simulink model "CubliParameterEstimation"  (R2015b)
settings: Solver=ode45  StartTime=0.0  StopTime=5  RelTol=1e-3
values from neighbouring files (symbols this model uses):
  B_f = b    [ParameterEstimationGradientCubli.m]    (also in costFunctionRecorder.m = 0.00608)
  g = 9.82    [ParameterEstimationGradientCubli.m]    (also in costFunctionRecorder.m)
  J_f = a    [ParameterEstimationGradientCubli.m]    (also in costFunctionRecorder.m = 0.0008)
  J_w = 0.601e-3    (= 0.000601)    [ParameterEstimationGradientCubli.m]    (also in costFunctionRecorder.m)
  l_f = 0.08498    [ParameterEstimationGradientCubli.m]    (also in costFunctionRecorder.m)
  l_w = 0.093    [ParameterEstimationGradientCubli.m]    (also in costFunctionRecorder.m)
  m_f = 0.77-m_w    (= 0.548)    [ParameterEstimationGradientCubli.m]    (also in costFunctionRecorder.m)
  m_w = 0.222    [ParameterEstimationGradientCubli.m]    (also in costFunctionRecorder.m)
settings Model: Creator=vniel  LastModifiedBy=USUARIO
settings DataIOCC: SaveFormat=Array  Refine=25
settings HardwareCC: ProdBitPerPointer=32  ProdLargestAtomicFloat=None  ProdIntDivRoundTo=Undefined  ProdEndianess=Unspecified  ProdWordSize=32  ProdHWDeviceType=32-bit Generic
settings GRTTargetCC: GeneratePreprocessorConditionals=Disable all
settings ConfigComp: CovModelRefEnable=Off

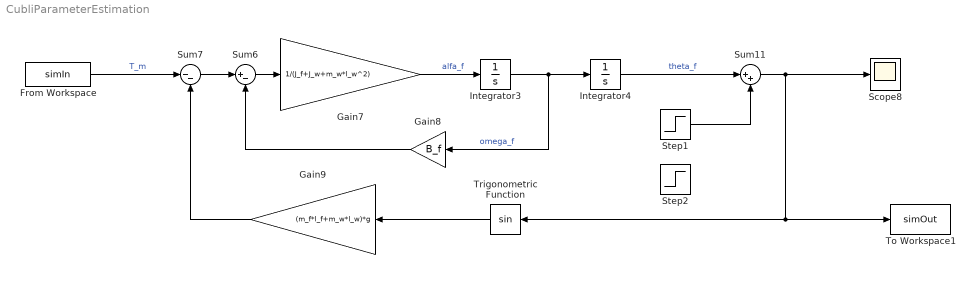
== system CubliParameterEstimation ==
  From Workspace : FromWorkspace  VariableName=simIn  SampleTime=0.01
  Gain7 : Gain  Gain=1/(J_f+J_w+m_w*l_w^2)
  Gain8 : Gain  Gain=B_f
  Gain9 : Gain  Gain=(m_f*l_f+m_w*l_w)*g
  Integrator3 : Integrator
  Integrator4 : Integrator
  Scope8 : Scope
  Step1 : Step  Time=0  After=0.1286  SampleTime=0
  Step2 : Step  Time=0  After=-0.09023  SampleTime=0
  Sum11 : Sum  Inputs=|++
  Sum6 : Sum  Inputs=|+-
  Sum7 : Sum  Inputs=|--
  To Workspace1 : ToWorkspace  VariableName=simOut  SampleTime=0.0025
      settings: MaxDataPoints=2000
  Trigonometric Function : Trigonometry
  wires:
  Gain7/1 -> Integrator3/1  "alfa_f"
  Integrator3/1 -> Gain8/1, Integrator4/1  "omega_f"
  Sum6/1 -> Gain7/1
  Sum7/1 -> Sum6/1
  Gain8/1 -> Sum6/2
  Gain9/1 -> Sum7/2
  Integrator4/1 -> Sum11/1  "theta_f"
  Trigonometric Function/1 -> Gain9/1
  From Workspace/1 -> Sum7/1  "T_m"
  Sum11/1 -> Trigonometric Function/1, To Workspace1/1, Scope8/1
  Step1/1 -> Sum11/2
